simulink model "EncoderReading"  (R2021b)
settings: Solver=FixedStepDiscrete  StartTime=0.0  StopTime=inf  FixedStep=0.001  RelTol=1e-3  EnableMultiTasking=on
undefined symbols (not defined in the file or in its folder): Ended, IO392, Single
libraries: speedgoatlib_IO191 x4, dspstat3 x4, speedgoatlib_fpga_quadrature x4, speedgoatlib_fpga x1
settings Model: SimulationMode=external  ExtModeEnableFloating=off  Creator=ET  LastModifiedBy=ET
settings SolverCC: ConcurrentTasks=on  AlgebraicLoopSolver=TrustRegion  PositivePriorityOrder=on  InsertRTBMode=Never (minimum delay)
settings DataIOCC: SaveFormat=Array  SaveState=on  SignalLoggingName=logsOut
settings OptimizationCC: BlockReduction=off  BooleanDataType=off  OptimizeBlockIOStorage=off  BufferReuse=off  GlobalBufferReuse=off  ExpressionFolding=off  LocalBlockOutputs=off  InitFltsAndDblsToZero=on  OptimizeDataStoreBuffers=off  BusAssignmentInplaceUpdate=off
settings DebuggingCC: SaveWithParameterizedLinksMsg=none  UnderspecifiedInitializationDetection=Classic  MergeDetectMultiDrivingBlocksExec=none  CheckExecutionContextPreStartOutputMsg=on  SignalResolutionControl=TryResolveAllWithWarning  TasksWithSamePriorityMsg=none  SFUnexpectedBacktrackingDiag=warning  SFNoUnconditionalDefaultTransitionDiag=warning  SFExecutionAtInitializationDiag=none  SFMachineParentedDataDiag=warning  ArithmeticOperatorsInVariantConditions=warning
settings HardwareCC: ProdBitPerLong=64  ProdLongLongMode=on  ProdHWDeviceType=Intel->x86-64 (Linux 64)
settings ModelReferenceCC: PropagateSignalLabelsOutOfModel=off
settings SFSimCC: SimUseLocalCustomCode=off  SimTargetLang=C++
settings RTWCC: Description=Simulink Real-Time  SystemTargetFile=slrealtime.tlc  TemplateMakefile=slrealtime_default_tmf  RTWUseLocalCustomCode=off  Toolchain=Simulink Real-Time Toolchain  BuildConfiguration=Faster Runs  CodeExecutionProfiling=on  TargetLang=C++
settings CodeAppCC: StateflowObjectComments=on
settings SimulinkRealTimeTargetCC: MATLABClassNameForMDSCustomization=Simulink.SoftwareTarget.GRTCustomization  UseGCCFastMath=on
settings ConfigComp: CovMetricSettings=dw  CovSaveCumulativeToWorkspaceVar=on  CovSaveSingleToWorkspaceVar=on  CovExternalEMLEnable=off  CovSFcnEnable=off

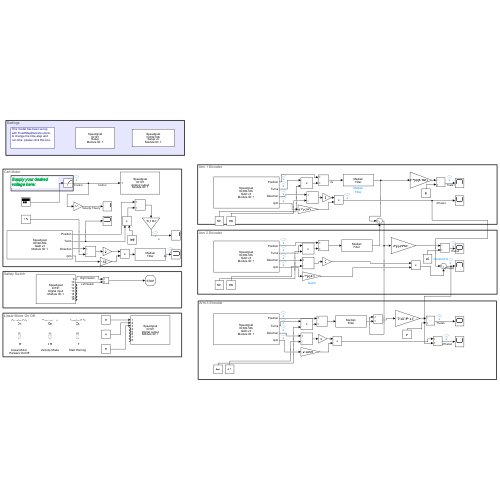
[thumbnail: Simulink's stored preview of the top-level diagram]
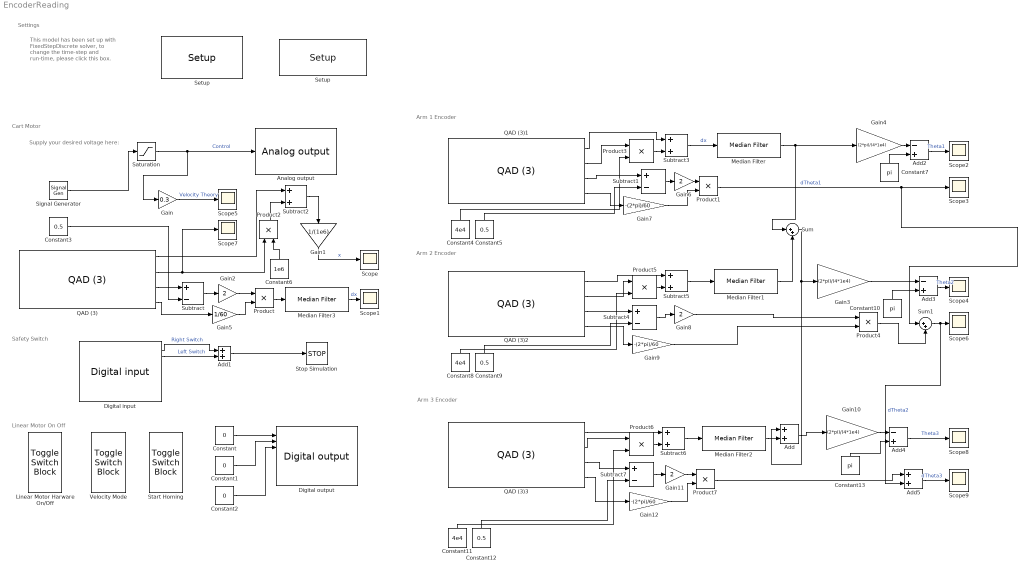
== system EncoderReading ==
  note: Arm 3 Encoder
  note: Supply your desired voltage here:
  note: This model has been set up with FixedStepDiscrete solver, to change the time-step and run-time, please click this box.
  note: Settings
  note: Linear Motor On Off
  note: Arm 1 Encoder
  note: Safety Switch
  note: Cart Motor
  note: Arm 2 Encoder
  Add : Sum
  Add1 : Sum
  Add2 : Sum  Inputs=-+
  Add3 : Sum  Inputs=-+
  Add4 : Sum  Inputs=-+
  Add5 : Sum
  "Analog output " : speedgoatlib_IO191/Analog output   parModuleId=1  parSampleTime=-1  parPciSlot=-1  parDacChannels=1  parModuleType=1  parDacRanges=4  parDacInitValues=0  parDacResets=1
      settings: SourceProductName=Simulink Real-Time: Speedgoat I/O Blockset
  Constant : Constant  Value=0
  Constant1 : Constant  Value=0
  Constant10 : Constant  Value=pi
  Constant11 : Constant  Value=4e4
  Constant{3,5,9,12} (4 alike) : Constant  Value=0.5
  Constant13 : Constant  Value=pi
  Constant2 : Constant  Value=0
  Constant4 : Constant  Value=4e4
  Constant6 : Constant  Value=1e6
  Constant7 : Constant  Value=pi
  Constant8 : Constant  Value=4e4
  "Digital input " : speedgoatlib_IO191/Digital input   parModuleId=1  parSampleTime=-1  parPciSlot=-1  parDiChannels=[9 10 11 12 13 14 15 16]
      settings: SourceProductName=Simulink Real-Time: Speedgoat I/O Blockset
  "Digital output " : speedgoatlib_IO191/Digital output   parModuleId=1  parSampleTime=-1  parPciSlot=-1  parDoChannels=[1 2 3 4 5 6 7 8]  parDoInitValues=[0 0 0 0 0 0 0 0]  parDoResets=[1 1 1 1 1 1 1 1]
      settings: SourceProductName=Simulink Real-Time: Speedgoat I/O Blockset
  Gain : Gain  Gain=0.3
  Gain1 : Gain  Gain=1/(1e6)
  Gain10 : Gain  Gain=(2*pi)/(4*1e4)
  Gain{2,6,8,11} (4 alike) : Gain  Gain=2
  Gain12 : Gain  Gain=-(2*pi)/60
  Gain3 : Gain  Gain=(2*pi)/(4*1e4)
  Gain4 : Gain  Gain=(2*pi)/(4*1e4)
  Gain5 : Gain  Gain=1/60
  Gain7 : Gain  Gain=-(2*pi)/60
  Gain9 : Gain  Gain=-(2*pi)/60
  Linear Motor Harware On/Off : ToggleSwitchBlock
      settings: Values={{'Off', 'On'}, [0 1]}
  Median Filter{,1..3} (4 alike) : dspstat3/Median Filter  WindowLength=3  SimulateUsing=Interpreted execution
      settings: SourceProductBaseCode=DS
  Product{,1..7} (8 alike) : Product
  QAD (3) : speedgoatlib_fpga_quadrature/QAD (3)  id=1  board=IO392-50k  chan=[4]  resetOnStart=on  ts=-1  pciSlot=-1  operatingMode=Quadrature decoder  indexControlMode=Ignore index  resolution=4x  stepsPerRevolution=1e6  latchMode=Disabled  interpolatePosition=on  invertAB=off  showClearPositionInput=off  showClearIndexFoundInput=off  showPositionOutput=on  showTurnOutput=on  showSpeedOutput=on  showDirectionOutput=on  showIndexFoundOutput=off
      settings: SourceProductName=Simulink Real-Time: Speedgoat I/O Blockset
  QAD (3)1 : speedgoatlib_fpga_quadrature/QAD (3)  id=1  board=IO392-50k  chan=[2]  resetOnStart=on  ts=-1  pciSlot=-1  operatingMode=Quadrature decoder  indexControlMode=Ignore index  resolution=4x  stepsPerRevolution=[40000]  latchMode=Disabled  interpolatePosition=on  invertAB=off  showClearPositionInput=off  showClearIndexFoundInput=off  showPositionOutput=on  showTurnOutput=on  showSpeedOutput=on  showDirectionOutput=on  showIndexFoundOutput=off
      settings: SourceProductName=Simulink Real-Time: Speedgoat I/O Blockset
  QAD (3)2 : speedgoatlib_fpga_quadrature/QAD (3)  id=1  board=IO392-50k  chan=[3]  resetOnStart=on  ts=-1  pciSlot=-1  operatingMode=Quadrature decoder  indexControlMode=Ignore index  resolution=4x  stepsPerRevolution=[40000]  latchMode=Disabled  interpolatePosition=on  invertAB=off  showClearPositionInput=off  showClearIndexFoundInput=off  showPositionOutput=on  showTurnOutput=on  showSpeedOutput=on  showDirectionOutput=on  showIndexFoundOutput=off
      settings: SourceProductName=Simulink Real-Time: Speedgoat I/O Blockset
  QAD (3)3 : speedgoatlib_fpga_quadrature/QAD (3)  id=1  board=IO392-50k  chan=[1]  resetOnStart=on  ts=-1  pciSlot=-1  operatingMode=Quadrature decoder  indexControlMode=Ignore index  resolution=4x  stepsPerRevolution=[40000]  latchMode=Disabled  interpolatePosition=on  invertAB=off  showClearPositionInput=off  showClearIndexFoundInput=off  showPositionOutput=on  showTurnOutput=on  showSpeedOutput=on  showDirectionOutput=on  showIndexFoundOutput=off
      settings: SourceProductName=Simulink Real-Time: Speedgoat I/O Blockset
  Saturation : Saturate  UpperLimit=10  LowerLimit=-10
  Scope{,1..9} (10 alike) : Scope
  Setup : speedgoatlib_fpga/Setup/Setup  board=IO392-50k  id=1  device_id=1  frontIO=None  rearIO=None  bitstreamFile=speedgoat_IO392_50k_CI_02385  rev=1.0  timestamp_string=09/08/21 13:42:38  fpgaFreq=75 MHz  fpgaTick=13.33 ns  ProgSpiFlash=off  ProgBPIFlash=off  pciSlot=-1  PullRPort0=pull-up 3.3V  VioPort0=3.3V  PullRPort1=pull-up 3.3V  VioPort1=3.3V  PullRPort2=pull-up 3.3V  VioPort2=3.3V  PullRPort3=pull-up 3.3V  VioPort3=3.3V  PullRPort4=pull-up 3.3V  VioPort4=3.3V  PullRPort5=pull-up 3.3V  VioPort5=3.3V  PullRPort6=pull-up 3.3V  VioPort6=3.3V  PullRPort15=pull-up 3.3V  PullRPort31=pull-up 3.3V  PullRPort47=pull-up 3.3V  PullRPort63=pull-up 3.3V
      settings: SourceProductName=Simulink Real-Time: Speedgoat I/O Blockset
  "Setup " : speedgoatlib_IO191/Setup   parModuleId=1  parPciSlot=-1  parTriggerSignal=TTL  parAdcChannels=[1 2]  parAdcRanges=[3 3]  parAdcChannel1=on  parAdcChannel2=on  parAdcChannel3=off  parAdcChannel4=off  parAdcChannel5=off  parAdcChannel6=off  parAdcChannel7=off  parAdcChannel8=off  parAdcMode=Single-Ended  parAdcRate=100000  parAdcRange11=+-10.24 V  parAdcRange21=+-24.576 V  parAdcRange12=+-10.24 V  parAdcRange22=+-24.576 V  parAdcRange13=+-10.24 V  parAdcRange23=+-24.576 V  parAdcRange14=+-10.24 V  parAdcRange24=+-24.576 V  parAdcRange15=+-10.24 V  parAdcRange25=+-24.576 V  parAdcRange16=+-10.24 V  parAdcRange26=+-24.576 V  parAdcRange17=+-10.24 V  parAdcRange27=+-24.576 V  parAdcRange18=+-10.24 V  parAdcRange28=+-24.576 V  parDacChannels=1  parDacChannel1=on  parDacChannel2=off  parDacChannel3=off  parDacChannel4=off  parDacMode=Single-Ended  parDacRanges=4  parDacInitValues=0  parDacResets=1  parDacRange1=+-10 V  parDacInitValue1=0  parDacReset1=on  parDacRange2=+-10 V  parDacInitValue2=0  parDacReset2=on  parDacRange3=+-10 V  parDacInitValue3=0  parDacReset3=on  parDacRange4=+-10 V  parDacInitValue4=0  parDacReset4=on  parDiChannels=[9 10 11 12 13 14 15 16]  parDoChannels=[1 2 3 4 5 6 7 8]  parDioFirstControl=1  parDioSecondControl=0  parDioChannel1=Out  parExtra1=I  parExtra2=I  parExtra3=I  parDioChannel2=In  parDioChannel3=In  parDioChannel4=In  parDioChannel5=In  parDioChannel6=In  parDioChannel7=In  parDioChannel8=In  parDioChannel9=In  parDoInitValues=[0 0 0 0]  parDoResets=[1 1 1 1]  parDoInitValue1=0  parDoReset1=on  parDoInitValue2=0  parDoReset2=on  parDoInitValue3=0  parDoReset3=on  parDoInitValue4=0  parDoReset4=on  parDoInitValue5=0  parDoReset5=on  parDoInitValue6=0  parDoReset6=on  parDoInitValue7=0  parDoReset7=on  parDoInitValue8=0  parDoReset8=on  parDoInitValue9=0  parDoReset9=on  parDoInitValue10=0  parDoReset10=on  parDoInitValue11=0  parDoReset11=on  parDoInitValue12=0  parDoReset12=on  parDoInitValue13=0  parDoReset13=on  parDoInitValue14=0  parDoReset14=on  parDoInitValue15=0  parDoReset15=on  parDoInitValue16=0  parDoReset16=on
      settings: SourceProductName=Simulink Real-Time: Speedgoat I/O Blockset
  Signal Generator : SignalGenerator  Amplitude=1.8  Frequency=20  Units=rad/sec
  Start Homing : ToggleSwitchBlock
      settings: Values={{'Off', 'On'}, [0 1]}
  Stop Simulation : Stop
  Subtract{,1,4,7} (4 alike) : Sum  Inputs=+-
  Subtract{2..3,5..6} (4 alike) : Sum
  Sum : Sum  Inputs=|++
  Sum1 : Sum  Inputs=|++
  Velocity Mode : ToggleSwitchBlock
      settings: Values={{'Off', 'On'}, [0 1]}
  wires:
  "Digital input "/1 -> Add1/1  "Right Switch"
  "Digital input "/2 -> Add1/2  "Left Switch"
  Constant/1 -> "Digital output "/1
  Constant1/1 -> "Digital output "/2
  Constant2/1 -> "Digital output "/3
  Gain/1 -> Scope5/1  "Velocity Theory"
  Saturation/1 -> Gain/1, "Analog output "/1  "Control"
  Add1/1 -> Stop Simulation/1
  QAD (3)/3 -> Subtract/1
  QAD (3)/4 -> Gain5/1
  Gain2/1 -> Product/1
  Subtract/1 -> Gain2/1
  Constant3/1 -> Subtract/2
  QAD (3)/2 -> Scope7/1, Product2/1
  QAD (3)/1 -> Subtract2/1
  Subtract2/1 -> Gain1/1
  Constant6/1 -> Product2/2
  Product2/1 -> Subtract2/2
  Gain1/1 -> Scope/1  "x"
  Gain5/1 -> Product/2
  Product/1 -> Median Filter3/1
  Median Filter3/1 -> Scope1/1  "dx"
  Gain6/1 -> Product1/1
  Product3/1 -> Subtract3/2
  Gain7/1 -> Product1/2
  QAD (3)1/1 -> Subtract3/1
  QAD (3)1/2 -> Product3/1
  Constant5/1 -> Subtract1/2
  Subtract1/1 -> Gain6/1
  Gain4/1 -> Add2/1
  QAD (3)1/3 -> Subtract1/1
  Add2/1 -> Scope2/1  "Theta1"
  Constant7/1 -> Add2/2
  QAD (3)1/4 -> Gain7/1
  Product1/1 -> Scope3/1, Sum1/1  "dTheta1"
  Constant4/1 -> Product3/2
  QAD (3)2/4 -> Gain9/1
  Gain3/1 -> Add3/1
  Constant10/1 -> Add3/2
  Constant8/1 -> Product5/2
  Constant9/1 -> Subtract4/2
  Gain9/1 -> Product4/2
  QAD (3)2/1 -> Subtract5/1
  QAD (3)2/2 -> Product5/1
  QAD (3)2/3 -> Subtract4/1
  Add3/1 -> Scope4/1  "Theta2"
  Gain8/1 -> Product4/1
  Product5/1 -> Subtract5/2
  Subtract4/1 -> Gain8/1
  Sum1/1 -> Add5/2, Scope6/1  "dTheta2"
  Product4/1 -> Sum1/2
  Subtract3/1 -> Median Filter/1  "dx"
  Signal Generator/1 -> Saturation/1
  Constant12/1 -> Subtract7/2
  Constant11/1 -> Product6/2
  QAD (3)3/1 -> Subtract6/1
  QAD (3)3/2 -> Product6/1
  Product6/1 -> Subtract6/2
  Subtract5/1 -> Median Filter1/1
  Sum/1 -> Add/1, Gain3/1
  Subtract6/1 -> Median Filter2/1
  Add/1 -> Gain10/1
  Gain10/1 -> Add4/1
  Constant13/1 -> Add4/2
  Add4/1 -> Scope8/1  "Theta3"
  QAD (3)3/3 -> Subtract7/1
  Subtract7/1 -> Gain11/1
  Gain11/1 -> Product7/1
  Gain12/1 -> Product7/2
  QAD (3)3/4 -> Gain12/1
  Product7/1 -> Add5/1
  Add5/1 -> Scope9/1  "dTheta3"
  Median Filter/1 -> Sum/1, Gain4/1
  Median Filter1/1 -> Sum/2
  Median Filter2/1 -> Add/2
